simulink model "Suspension"  (R2019b)
settings: Solver=VariableStepAuto  StartTime=0.0  StopTime=10.0  RelTol=1e-3
values from neighbouring files (symbols this model uses):
  cfs = 1290    [Suspension_parameter.m]
  cft = 1000    [Suspension_parameter.m]
  crs = 1620    [Suspension_parameter.m]
  crt = 1000    [Suspension_parameter.m]
  iyy = 2460    [Suspension_parameter.m]
  kfs = 19960    [Suspension_parameter.m]
  kft = 175500    [Suspension_parameter.m]
  krs = 17500    [Suspension_parameter.m]
  krt = 175500    [Suspension_parameter.m]
  lf = 2.3    [Suspension_parameter.m]
  lr = 2.3    [Suspension_parameter.m]
  mc = 700    [Suspension_parameter.m]
  mf = 40    [Suspension_parameter.m]
  mr = 35.5    [Suspension_parameter.m]
libraries: simulink x4
(part 1 of 2)
settings Model: Creator=홍승표  LastModifiedBy=홍승표

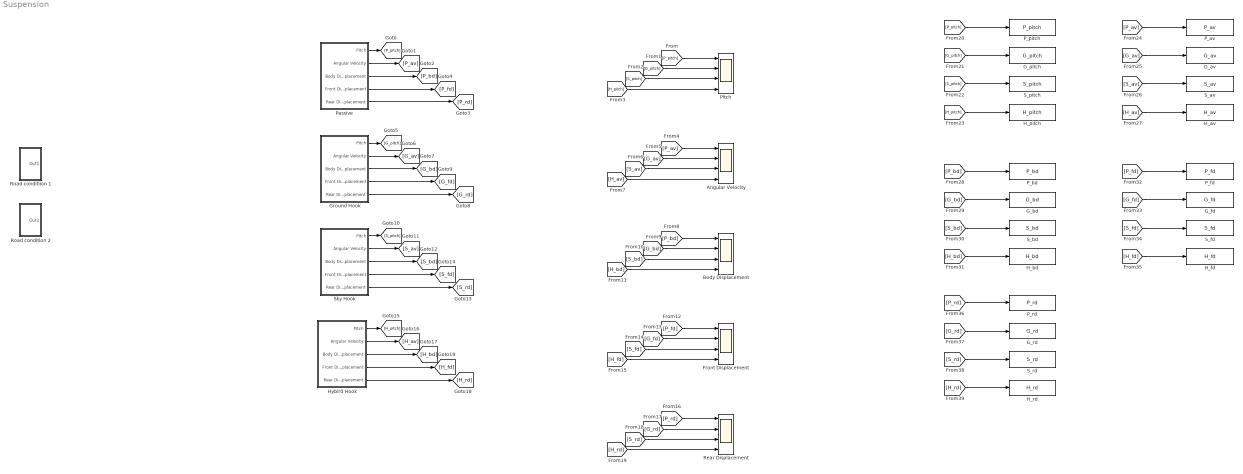
== system Suspension ==
  Angular Velocity : Scope  NumInputPorts=4
  Body Displacement : Scope  NumInputPorts=4
  Front Displacement : Scope  NumInputPorts=4
  G_av : ToWorkspace  VariableName=G_av  SampleTime=-1
  G_bd : ToWorkspace  VariableName=G_bd  SampleTime=-1
  G_fd : ToWorkspace  VariableName=G_fd  SampleTime=-1
  G_pitch : ToWorkspace  VariableName=G_pitch  SampleTime=-1
  G_rd : ToWorkspace  VariableName=G_rd  SampleTime=-1
  Ground Hook : Subsystem
  H_av : ToWorkspace  VariableName=H_av  SampleTime=-1
  H_bd : ToWorkspace  VariableName=H_bd  SampleTime=-1
  H_fd : ToWorkspace  VariableName=H_fd  SampleTime=-1
  H_pitch : ToWorkspace  VariableName=H_pitch  SampleTime=-1
  H_rd : ToWorkspace  VariableName=H_rd  SampleTime=-1
  Hybird Hook : Subsystem
  P_av : ToWorkspace  VariableName=P_av  SampleTime=-1
  P_bd : ToWorkspace  VariableName=P_bd  SampleTime=-1
  P_fd : ToWorkspace  VariableName=P_fd  SampleTime=-1
  P_pitch : ToWorkspace  VariableName=P_pitch  SampleTime=-1
  P_rd : ToWorkspace  VariableName=P_rd  SampleTime=-1
  Passive : Subsystem
  Pitch : Scope  NumInputPorts=4
  Rear Displacement : Scope  NumInputPorts=4
  Road conditiion 1 : Subsystem
  "Road condition 2 " : Subsystem
  S_av : ToWorkspace  VariableName=S_av  SampleTime=-1
  S_bd : ToWorkspace  VariableName=S_bd  SampleTime=-1
  S_fd : ToWorkspace  VariableName=S_fd  SampleTime=-1
  S_pitch : ToWorkspace  VariableName=S_pitch  SampleTime=-1
  S_rd : ToWorkspace  VariableName=S_rd  SampleTime=-1
  Sky Hook : Subsystem
  wires:
  Passive/1(Pitch) -> [P_pitch]
  Passive/2(Angular Velocity) -> [P_av]
  Passive/3(Body Displacement) -> [P_bd]
  Passive/4(Front Displacement) -> [P_fd]
  Passive/5(Rear Displacement) -> [P_rd]
  Ground Hook/2(Angular Velocity) -> [G_av]
  Ground Hook/5(Rear Displacement) -> [G_rd]
  Ground Hook/3(Body Displacement) -> [G_bd]
  Ground Hook/4(Front Displacement) -> [G_fd]
  Ground Hook/1(Pitch) -> [G_pitch]
  Sky Hook/4(Front Displacement) -> [S_fd]
  Sky Hook/1(Pitch) -> [S_pitch]
  Sky Hook/5(Rear Displacement) -> [S_rd]
  Sky Hook/2(Angular Velocity) -> [S_av]
  Sky Hook/3(Body Displacement) -> [S_bd]
  Hybird Hook/4(Front Displacement) -> [H_fd]
  Hybird Hook/1(Pitch) -> [H_pitch]
  Hybird Hook/5(Rear Displacement) -> [H_rd]
  Hybird Hook/2(Angular Velocity) -> [H_av]
  Hybird Hook/3(Body Displacement) -> [H_bd]
  [P_pitch] -> Pitch/1
  [G_pitch] -> Pitch/2
  [S_pitch] -> Pitch/3
  [H_pitch] -> Pitch/4
  [S_av] -> Angular Velocity/3
  [G_av] -> Angular Velocity/2
  [P_av] -> Angular Velocity/1
  [H_av] -> Angular Velocity/4
  [S_bd] -> Body Displacement/3
  [G_bd] -> Body Displacement/2
  [P_bd] -> Body Displacement/1
  [H_bd] -> Body Displacement/4
  [S_fd] -> Front Displacement/3
  [G_fd] -> Front Displacement/2
  [P_fd] -> Front Displacement/1
  [H_fd] -> Front Displacement/4
  [S_rd] -> Rear Displacement/3
  [G_rd] -> Rear Displacement/2
  [P_rd] -> Rear Displacement/1
  [H_rd] -> Rear Displacement/4
  [P_pitch] -> P_pitch/1
  [G_pitch] -> G_pitch/1
  [S_pitch] -> S_pitch/1
  [H_pitch] -> H_pitch/1
  [H_av] -> H_av/1
  [S_av] -> S_av/1
  [P_av] -> P_av/1
  [G_av] -> G_av/1
  [G_bd] -> G_bd/1
  [S_bd] -> S_bd/1
  [P_bd] -> P_bd/1
  [H_bd] -> H_bd/1
  [S_fd] -> S_fd/1
  [G_fd] -> G_fd/1
  [P_fd] -> P_fd/1
  [H_fd] -> H_fd/1
  [S_rd] -> S_rd/1
  [G_rd] -> G_rd/1
  [P_rd] -> P_rd/1
  [H_rd] -> H_rd/1

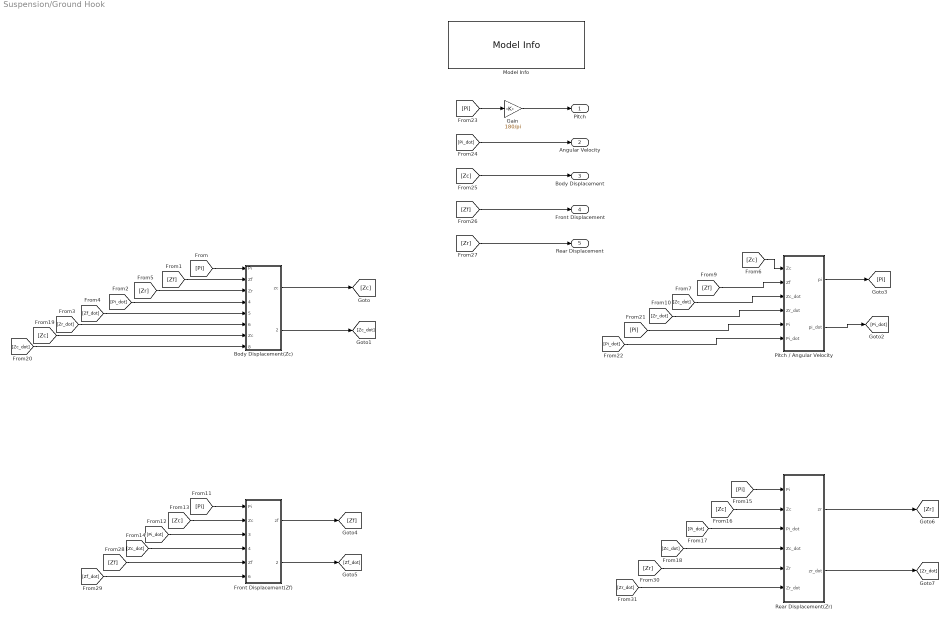
== system Suspension/Ground Hook ==
  Body Displacement(Zc) : Subsystem
  Front Displacement(Zf) : Subsystem
  Gain : Gain  Gain=180/pi
  Model Info : simulink/Model-Wide Utilities/Model Info  Frame=on  DisplayStringWithTags=Ground  HorizontalTextAlignment=Center  LeftAlignmentValue=0.5
  Pitch / Angular Velocity : Subsystem
  Rear Displacement(Zr) : Subsystem
  Pitch : Outport
  Angular Velocity : Outport  Port=2
  Body Displacement : Outport  Port=3
  Front Displacement : Outport  Port=4
  Rear Displacement : Outport  Port=5
  wires:
  [Pi_dot] -> Body Displacement(Zc)/4(Pi_dot)
  [Pi] -> Gain/1
  Front Displacement(Zf)/1(zf) -> [Zf]
  [Pi] -> Front Displacement(Zf)/1(Pi)
  Body Displacement(Zc)/1(zc) -> [Zc]
  [Pi_dot] -> Angular Velocity/1
  [Pi_dot] -> Rear Displacement(Zr)/3(Pi_dot)
  [Zr] -> Body Displacement(Zc)/3(Zr)
  [Zc_dot] -> Rear Displacement(Zr)/4(Zc_dot)
  [Zc] -> Body Displacement/1
  [Zr_dot] -> Body Displacement(Zc)/6(Zr_dot)
  Rear Displacement(Zr)/2(zr_dot) -> [Zr_dot]
  [Pi] -> Rear Displacement(Zr)/1(Pi)
  [Zf] -> Body Displacement(Zc)/2(Zf)
  [Zf_dot] -> Body Displacement(Zc)/5(Zf_dot)
  [Zc_dot] -> Front Displacement(Zf)/4(Zc_dot)
  Rear Displacement(Zr)/1(zr) -> [Zr]
  [Zc] -> Front Displacement(Zf)/2(Zc)
  [Zr] -> Rear Displacement/1
  Body Displacement(Zc)/2(zc_dot) -> [Zc_dot]
  Gain/1 -> Pitch/1
  [Zc] -> Rear Displacement(Zr)/2(Zc)
  [Zf] -> Front Displacement/1
  [Pi_dot] -> Front Displacement(Zf)/3(Pi_dot)
  Front Displacement(Zf)/2(zf_dot) -> [Zf_dot]
  [Pi] -> Body Displacement(Zc)/1(Pi)
  [Zc] -> Body Displacement(Zc)/7(Zc)
  [Zc_dot] -> Body Displacement(Zc)/8(Zc_dot)
  [Zf] -> Front Displacement(Zf)/5(Zf)
  [Zf_dot] -> Front Displacement(Zf)/6(Zf_dot)
  [Zr] -> Rear Displacement(Zr)/5(Zr)
  [Zr_dot] -> Rear Displacement(Zr)/6(Zr_dot)
  Pitch / Angular Velocity/1(pi) -> [Pi]
  [Pi] -> Pitch / Angular Velocity/5(Pi)
  [Zf] -> Pitch / Angular Velocity/2(Zf)
  [Zc_dot] -> Pitch / Angular Velocity/3(Zc_dot)
  [Zr_dot] -> Pitch / Angular Velocity/4(Zr_dot)
  Pitch / Angular Velocity/2(pi_dot) -> [Pi_dot]
  [Pi_dot] -> Pitch / Angular Velocity/6(Pi_dot)
  [Zc] -> Pitch / Angular Velocity/1(Zc)

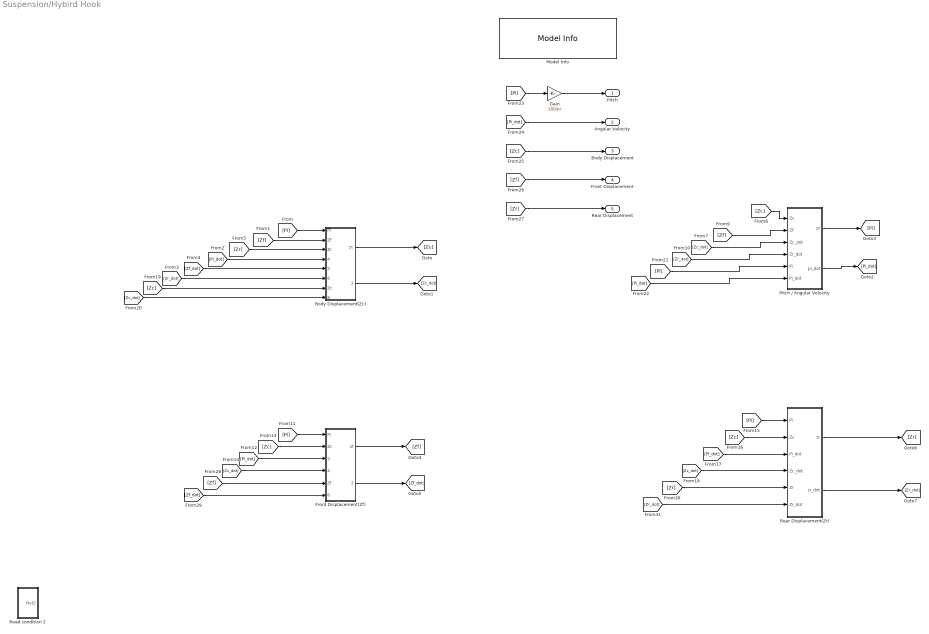
== system Suspension/Hybird Hook ==
  Body Displacement(Zc) : Subsystem
  Front Displacement(Zf) : Subsystem
  Gain : Gain  Gain=180/pi
  Model Info : simulink/Model-Wide Utilities/Model Info  Frame=on  DisplayStringWithTags=Hybrid  HorizontalTextAlignment=Center  LeftAlignmentValue=0.5
  Pitch / Angular Velocity : Subsystem
  Rear Displacement(Zr) : Subsystem
  "Road condition 2 " : Subsystem
  Pitch : Outport
  Angular Velocity : Outport  Port=2
  Body Displacement : Outport  Port=3
  Front Displacement : Outport  Port=4
  Rear Displacement : Outport  Port=5
  wires:
  [Pi_dot] -> Body Displacement(Zc)/4(Pi_dot)
  [Pi] -> Gain/1
  Front Displacement(Zf)/1(zf) -> [Zf]
  [Pi] -> Front Displacement(Zf)/1(Pi)
  Body Displacement(Zc)/1(zc) -> [Zc]
  [Pi_dot] -> Angular Velocity/1
  [Pi_dot] -> Rear Displacement(Zr)/3(Pi_dot)
  [Zr] -> Body Displacement(Zc)/3(Zr)
  [Zc_dot] -> Rear Displacement(Zr)/4(Zc_dot)
  [Zc] -> Body Displacement/1
  [Zr_dot] -> Body Displacement(Zc)/6(Zr_dot)
  Rear Displacement(Zr)/2(zr_dot) -> [Zr_dot]
  [Pi] -> Rear Displacement(Zr)/1(Pi)
  [Zf] -> Body Displacement(Zc)/2(Zf)
  [Zf_dot] -> Body Displacement(Zc)/5(Zf_dot)
  [Zc_dot] -> Front Displacement(Zf)/4(Zc_dot)
  Rear Displacement(Zr)/1(zr) -> [Zr]
  [Zc] -> Front Displacement(Zf)/2(Zc)
  [Zr] -> Rear Displacement/1
  Body Displacement(Zc)/2(zc_dot) -> [Zc_dot]
  Gain/1 -> Pitch/1
  [Zc] -> Rear Displacement(Zr)/2(Zc)
  [Zf] -> Front Displacement/1
  [Pi_dot] -> Front Displacement(Zf)/3(Pi_dot)
  Front Displacement(Zf)/2(zf_dot) -> [Zf_dot]
  [Pi] -> Body Displacement(Zc)/1(Pi)
  [Zc] -> Body Displacement(Zc)/7(Zc)
  [Zc_dot] -> Body Displacement(Zc)/8(Zc_dot)
  [Zf] -> Front Displacement(Zf)/5(Zf)
  [Zf_dot] -> Front Displacement(Zf)/6(Zf_dot)
  [Zr] -> Rear Displacement(Zr)/5(Zr)
  [Zr_dot] -> Rear Displacement(Zr)/6(Zr_dot)
  Pitch / Angular Velocity/1(pi) -> [Pi]
  [Pi] -> Pitch / Angular Velocity/5(Pi)
  [Zf] -> Pitch / Angular Velocity/2(Zf)
  [Zc_dot] -> Pitch / Angular Velocity/3(Zc_dot)
  [Zr_dot] -> Pitch / Angular Velocity/4(Zr_dot)
  Pitch / Angular Velocity/2(pi_dot) -> [Pi_dot]
  [Pi_dot] -> Pitch / Angular Velocity/6(Pi_dot)
  [Zc] -> Pitch / Angular Velocity/1(Zc)

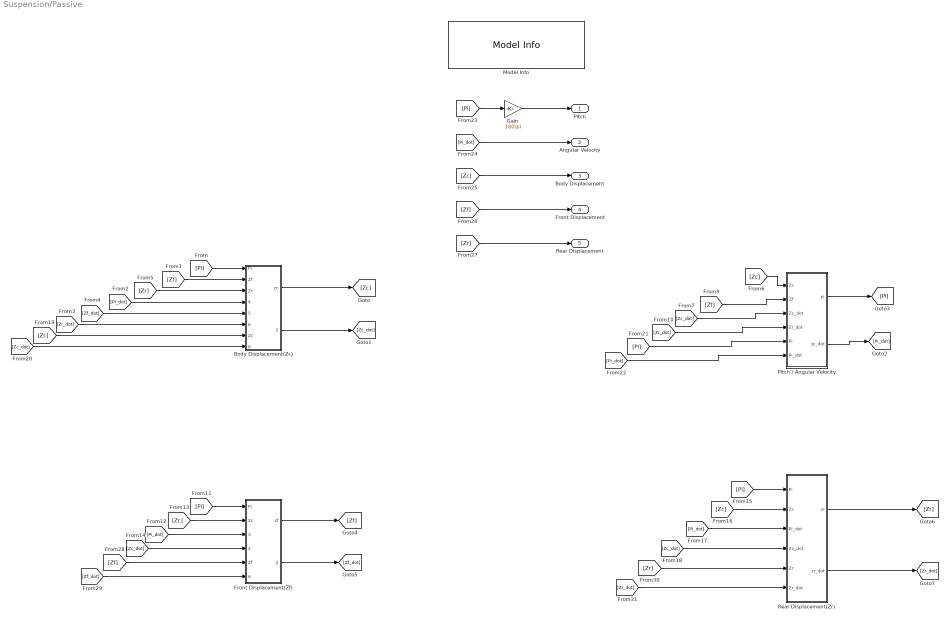
== system Suspension/Passive ==
  Body Displacement(Zc) : Subsystem
  Front Displacement(Zf) : Subsystem
  Gain : Gain  Gain=180/pi
  Model Info : simulink/Model-Wide Utilities/Model Info  Frame=on  DisplayStringWithTags=Passive  HorizontalTextAlignment=Center  LeftAlignmentValue=0.5
  Pitch / Angular Velocity : Subsystem
  Rear Displacement(Zr) : Subsystem
  Pitch : Outport
  Angular Velocity : Outport  Port=2
  Body Displacement : Outport  Port=3
  Front Displacement : Outport  Port=4
  Rear Displacement : Outport  Port=5
  wires:
  [Pi_dot] -> Body Displacement(Zc)/4(Pi_dot)
  [Pi] -> Gain/1
  Front Displacement(Zf)/1(zf) -> [Zf]
  [Pi] -> Front Displacement(Zf)/1(Pi)
  Body Displacement(Zc)/1(zc) -> [Zc]
  [Pi_dot] -> Angular Velocity/1
  [Pi_dot] -> Rear Displacement(Zr)/3(Pi_dot)
  [Zr] -> Body Displacement(Zc)/3(Zr)
  [Zc_dot] -> Rear Displacement(Zr)/4(Zc_dot)
  [Zc] -> Body Displacement/1
  [Zr_dot] -> Pitch / Angular Velocity/4(Zr_dot)
  [Zr_dot] -> Body Displacement(Zc)/6(Zr_dot)
  Rear Displacement(Zr)/2(zr_dot) -> [Zr_dot]
  [Pi] -> Rear Displacement(Zr)/1(Pi)
  [Zf] -> Body Displacement(Zc)/2(Zf)
  Pitch / Angular Velocity/1(pi) -> [Pi]
  [Zf_dot] -> Body Displacement(Zc)/5(Zf_dot)
  [Zc_dot] -> Front Displacement(Zf)/4(Zc_dot)
  Rear Displacement(Zr)/1(zr) -> [Zr]
  [Zc] -> Front Displacement(Zf)/2(Zc)
  [Zc] -> Pitch / Angular Velocity/1(Zc)
  [Zr] -> Rear Displacement/1
  Body Displacement(Zc)/2(zc_dot) -> [Zc_dot]
  Gain/1 -> Pitch/1
  [Zf] -> Pitch / Angular Velocity/2(Zf)
  [Zc_dot] -> Pitch / Angular Velocity/3(Zc_dot)
  [Zc] -> Rear Displacement(Zr)/2(Zc)
  [Zf] -> Front Displacement/1
  [Pi_dot] -> Front Displacement(Zf)/3(Pi_dot)
  Pitch / Angular Velocity/2(pi_dot) -> [Pi_dot]
  Front Displacement(Zf)/2(zf_dot) -> [Zf_dot]
  [Pi] -> Body Displacement(Zc)/1(Pi)
  [Zc] -> Body Displacement(Zc)/7(Zc)
  [Zc_dot] -> Body Displacement(Zc)/8(Zc_dot)
  [Pi] -> Pitch / Angular Velocity/5(Pi)
  [Pi_dot] -> Pitch / Angular Velocity/6(Pi_dot)
  [Zf] -> Front Displacement(Zf)/5(Zf)
  [Zf_dot] -> Front Displacement(Zf)/6(Zf_dot)
  [Zr] -> Rear Displacement(Zr)/5(Zr)
  [Zr_dot] -> Rear Displacement(Zr)/6(Zr_dot)

== system Suspension/Road conditiion 1 ==
  Gain : Gain
  Product : Product  Inputs=3
  Scope : Scope
  Signal Generator : SignalGenerator  Amplitude=0.15  Frequency=1.852  Units=rad/sec
  Step : Step  SampleTime=1.08
  Step1 : Step  Before=1  After=0  SampleTime=1.35
  Out1 : Outport
  wires:
  Gain/1 -> Out1/1
  Step1/1 -> Product/3
  Product/1 -> Gain/1, Scope/1
  Step/1 -> Product/2
  Signal Generator/1 -> Product/1

== system Suspension/Road condition 2  ==
  Product : Product  Inputs=3
  Saturation : Saturate  LowerLimit=0
  Scope : Scope
  Scope1 : Scope  NumInputPorts=3
  Signal Generator : SignalGenerator  Amplitude=0.15  Frequency=1.852
  Step : Step  SampleTime=1.08
  Step1 : Step  Before=1  After=0  SampleTime=4
  Out2 : Outport
  wires:
  Signal Generator/1 -> Scope1/1, Product/1
  Product/1 -> Out2/1, Saturation/1
  Step/1 -> Scope1/2, Product/2
  Step1/1 -> Scope1/3, Product/3
  Saturation/1 -> Scope/1

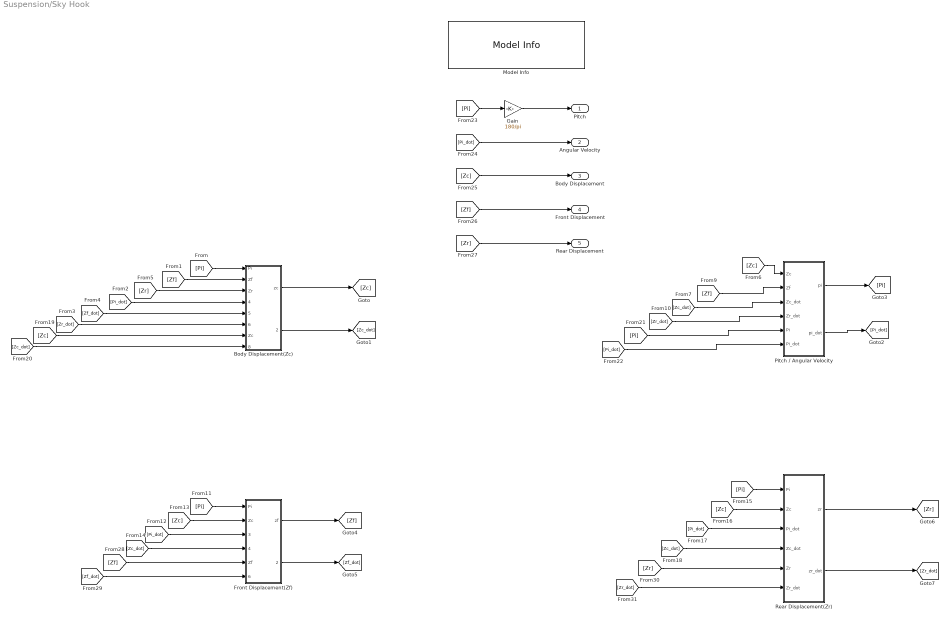
== system Suspension/Sky Hook ==
  Body Displacement(Zc) : Subsystem
  Front Displacement(Zf) : Subsystem
  Gain : Gain  Gain=180/pi
  Model Info : simulink/Model-Wide Utilities/Model Info  Frame=on  DisplayStringWithTags=Sky  HorizontalTextAlignment=Center  LeftAlignmentValue=0.5
  Pitch / Angular Velocity : Subsystem
  Rear Displacement(Zr) : Subsystem
  Pitch : Outport
  Angular Velocity : Outport  Port=2
  Body Displacement : Outport  Port=3
  Front Displacement : Outport  Port=4
  Rear Displacement : Outport  Port=5
  wires:
  [Pi_dot] -> Body Displacement(Zc)/4(Pi_dot)
  [Pi] -> Gain/1
  Front Displacement(Zf)/1(zf) -> [Zf]
  [Pi] -> Front Displacement(Zf)/1(Pi)
  Body Displacement(Zc)/1(zc) -> [Zc]
  [Pi_dot] -> Angular Velocity/1
  [Pi_dot] -> Rear Displacement(Zr)/3(Pi_dot)
  [Zr] -> Body Displacement(Zc)/3(Zr)
  [Zc_dot] -> Rear Displacement(Zr)/4(Zc_dot)
  [Zc] -> Body Displacement/1
  [Zr_dot] -> Body Displacement(Zc)/6(Zr_dot)
  Rear Displacement(Zr)/2(zr_dot) -> [Zr_dot]
  [Pi] -> Rear Displacement(Zr)/1(Pi)
  [Zf] -> Body Displacement(Zc)/2(Zf)
  [Zf_dot] -> Body Displacement(Zc)/5(Zf_dot)
  [Zc_dot] -> Front Displacement(Zf)/4(Zc_dot)
  Rear Displacement(Zr)/1(zr) -> [Zr]
  [Zc] -> Front Displacement(Zf)/2(Zc)
  [Zr] -> Rear Displacement/1
  Body Displacement(Zc)/2(zc_dot) -> [Zc_dot]
  Gain/1 -> Pitch/1
  [Zc] -> Rear Displacement(Zr)/2(Zc)
  [Zf] -> Front Displacement/1
  [Pi_dot] -> Front Displacement(Zf)/3(Pi_dot)
  Front Displacement(Zf)/2(zf_dot) -> [Zf_dot]
  [Pi] -> Body Displacement(Zc)/1(Pi)
  [Zc] -> Body Displacement(Zc)/7(Zc)
  [Zc_dot] -> Body Displacement(Zc)/8(Zc_dot)
  [Zf] -> Front Displacement(Zf)/5(Zf)
  [Zf_dot] -> Front Displacement(Zf)/6(Zf_dot)
  [Zr] -> Rear Displacement(Zr)/5(Zr)
  [Zr_dot] -> Rear Displacement(Zr)/6(Zr_dot)
  Pitch / Angular Velocity/1(pi) -> [Pi]
  [Pi] -> Pitch / Angular Velocity/5(Pi)
  [Zf] -> Pitch / Angular Velocity/2(Zf)
  [Zc_dot] -> Pitch / Angular Velocity/3(Zc_dot)
  [Zr_dot] -> Pitch / Angular Velocity/4(Zr_dot)
  Pitch / Angular Velocity/2(pi_dot) -> [Pi_dot]
  [Pi_dot] -> Pitch / Angular Velocity/6(Pi_dot)
  [Zc] -> Pitch / Angular Velocity/1(Zc)

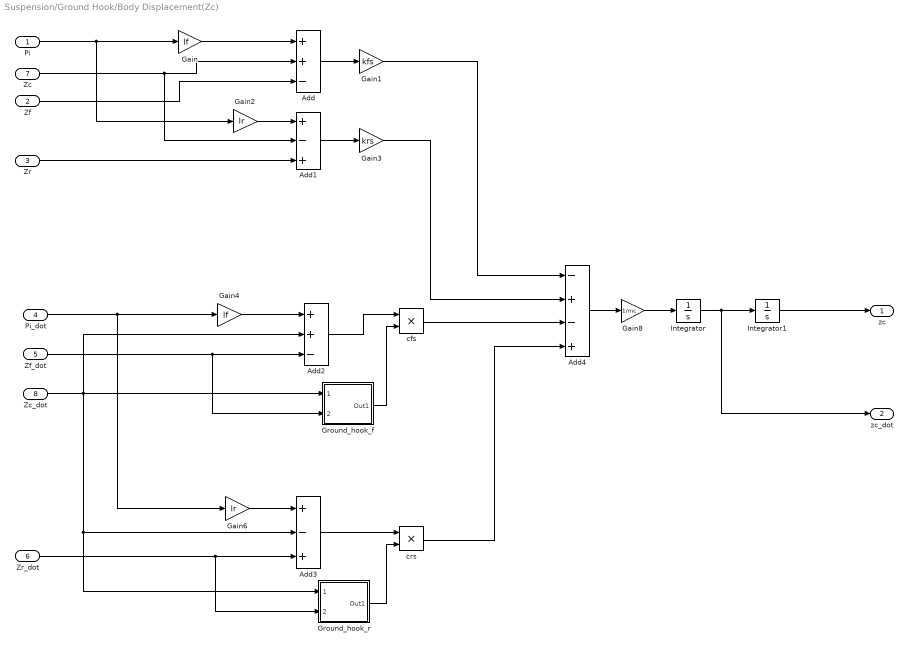
== system Suspension/Ground Hook/Body Displacement(Zc) ==
  Pi : Inport
  Zf : Inport  Port=2
  Zr : Inport  Port=3
  Pi_dot : Inport  Port=4
  Zf_dot : Inport  Port=5
  Zr_dot : Inport  Port=6
  Zc : Inport  Port=7
  Zc_dot : Inport  Port=8
  Add : Sum  Inputs=++-
  Add1 : Sum  Inputs=+-+
  Add2 : Sum  Inputs=++-
  Add3 : Sum  Inputs=+-+
  Add4 : Sum  Inputs=-+-+
  Gain : Gain  Gain=lf
  Gain1 : Gain  Gain=kfs
  Gain2 : Gain  Gain=lr
  Gain3 : Gain  Gain=krs
  Gain4 : Gain  Gain=lf
  Gain6 : Gain  Gain=lr
  Gain8 : Gain  Gain=1/mc
  Ground_hook_f : Subsystem
  Ground_hook_r : Subsystem
  Integrator : Integrator
  Integrator1 : Integrator
  cfs : Product
  crs : Product
  zc : Outport
  zc_dot : Outport  Port=2
  wires:
  Add/1 -> Gain1/1
  Add2/1 -> cfs/1
  Pi/1 -> Gain2/1, Gain/1
  Add4/1 -> Gain8/1
  Zr_dot/1 -> Ground_hook_r/2(Zr_dot), Add3/3
  Integrator/1 -> zc_dot/1, Integrator1/1
  Gain2/1 -> Add1/1
  Gain1/1 -> Add4/1
  Gain/1 -> Add/1
  Integrator1/1 -> zc/1
  crs/1 -> Add4/4
  Zr/1 -> Add1/3
  Add3/1 -> crs/1
  Zf_dot/1 -> Ground_hook_f/2(Zf_dot), Add2/3
  Gain6/1 -> Add3/1
  Gain3/1 -> Add4/2
  Pi_dot/1 -> Gain6/1, Gain4/1
  Gain4/1 -> Add2/1
  Add1/1 -> Gain3/1
  cfs/1 -> Add4/3
  Zf/1 -> Add/3
  Gain8/1 -> Integrator/1
  Ground_hook_f/1(Out1) -> cfs/2
  Ground_hook_r/1(Out1) -> crs/2
  Zc/1 -> Add1/2, Add/2
  Zc_dot/1 -> Add3/2, Ground_hook_r/1(Zc_dot), Ground_hook_f/1(Zc_dot), Add2/2

== system Suspension/Ground Hook/Front Displacement(Zf) ==
  Pi : Inport
  Zc : Inport  Port=2
  Pi_dot : Inport  Port=3
  Zc_dot : Inport  Port=4
  Zf : Inport  Port=5
  Zf_dot : Inport  Port=6
  Add10 : Sum  Inputs=++-
  Add11 : Sum  Inputs=++-
  Add12 : Sum  Inputs=+-
  Add13 : Sum  Inputs=+-
  Add14 : Sum  Inputs=++--
  Derivative : Derivative
  Gain22 : Gain  Gain=lf
  Gain23 : Gain  Gain=kfs
  Gain24 : Gain  Gain=lf
  Gain26 : Gain  Gain=kft
  Gain27 : Gain  Gain=cft
  Gain28 : Gain  Gain=1/mf
  Ground_hook_f : Subsystem
  Integrator4 : Integrator
  Integrator5 : Integrator
  Road conditiion 1 : Subsystem
  "Road condition 2 " : Subsystem
  cfs : Product
  zf : Outport
  zf_dot : Outport  Port=2
  wires:
  Gain28/1 -> Integrator4/1
  cfs/1 -> Add14/2
  Gain27/1 -> Add14/4
  Integrator4/1 -> zf_dot/1, Integrator5/1
  Add10/1 -> Gain23/1
  Integrator5/1 -> zf/1
  Gain24/1 -> Add11/1
  Gain23/1 -> Add14/1
  Add12/1 -> Gain27/1
  Gain26/1 -> Add14/3
  Gain22/1 -> Add10/1
  Add13/1 -> Gain26/1
  Add11/1 -> cfs/1
  Add14/1 -> Gain28/1
  Pi/1 -> Gain22/1
  Pi_dot/1 -> Gain24/1
  Zc/1 -> Add10/2
  Zc_dot/1 -> Ground_hook_f/1(Zc_dot), Add11/2
  Ground_hook_f/1(Out1) -> cfs/2
  Road conditiion 1/1(Out1) -> Add13/2, Derivative/1
  Derivative/1 -> Add12/2
  Zf/1 -> Add13/1, Add10/3
  Zf_dot/1 -> Add12/1, Add11/3, Ground_hook_f/2(Zf_dot)

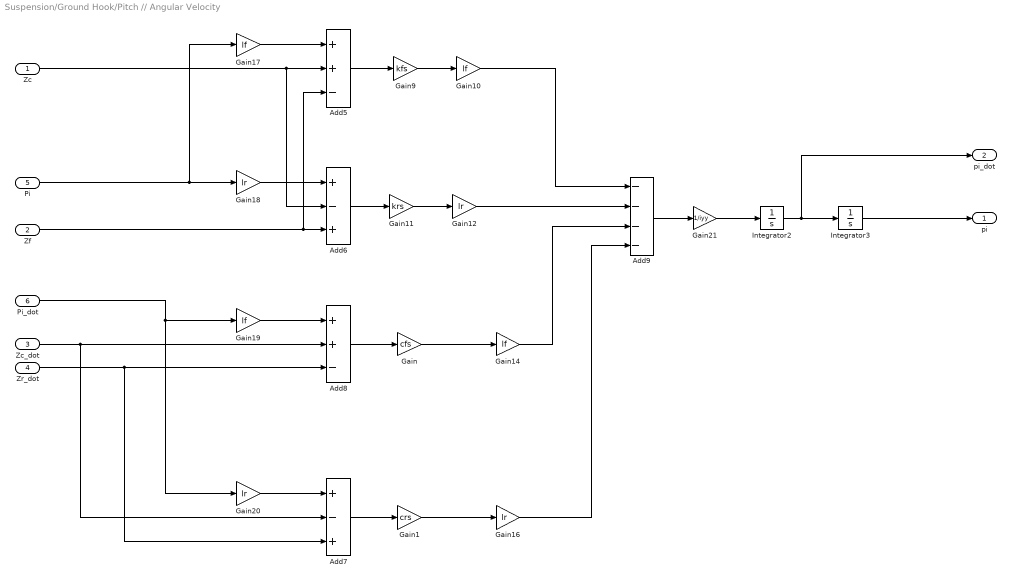
== system Suspension/Ground Hook/Pitch // Angular Velocity ==
  Zc : Inport
  Zf : Inport  Port=2
  Zc_dot : Inport  Port=3
  Zr_dot : Inport  Port=4
  Pi : Inport  Port=5
  Pi_dot : Inport  Port=6
  Add5 : Sum  Inputs=++-
  Add6 : Sum  Inputs=+-+
  Add7 : Sum  Inputs=+-+
  Add8 : Sum  Inputs=++-
  Add9 : Sum  Inputs=----
  Gain : Gain  Gain=cfs
  Gain1 : Gain  Gain=crs
  Gain{10,14,17,19} (4 alike) : Gain  Gain=lf
  Gain11 : Gain  Gain=krs
  Gain{12,16,18,20} (4 alike) : Gain  Gain=lr
  Gain21 : Gain  Gain=1/iyy
  Gain9 : Gain  Gain=kfs
  Integrator2 : Integrator
  Integrator3 : Integrator
  pi : Outport
  pi_dot : Outport  Port=2
  wires:
  Integrator3/1 -> pi/1
  Gain20/1 -> Add7/1
  Gain11/1 -> Gain12/1
  Gain9/1 -> Gain10/1
  Gain12/1 -> Add9/2
  Zc/1 -> Add6/2, Add5/2
  Add9/1 -> Gain21/1
  Gain17/1 -> Add5/1
  Zc_dot/1 -> Add7/2, Add8/2
  Gain16/1 -> Add9/4
  Zr_dot/1 -> Add7/3, Add8/3
  Integrator2/1 -> pi_dot/1, Integrator3/1
  Gain18/1 -> Add6/1
  Gain19/1 -> Add8/1
  Gain21/1 -> Integrator2/1
  Gain14/1 -> Add9/3
  Gain10/1 -> Add9/1
  Add5/1 -> Gain9/1
  Add6/1 -> Gain11/1
  Zf/1 -> Add5/3, Add6/3
  Pi_dot/1 -> Gain20/1, Gain19/1
  Pi/1 -> Gain17/1, Gain18/1
  Add8/1 -> Gain/1
  Gain/1 -> Gain14/1
  Add7/1 -> Gain1/1
  Gain1/1 -> Gain16/1

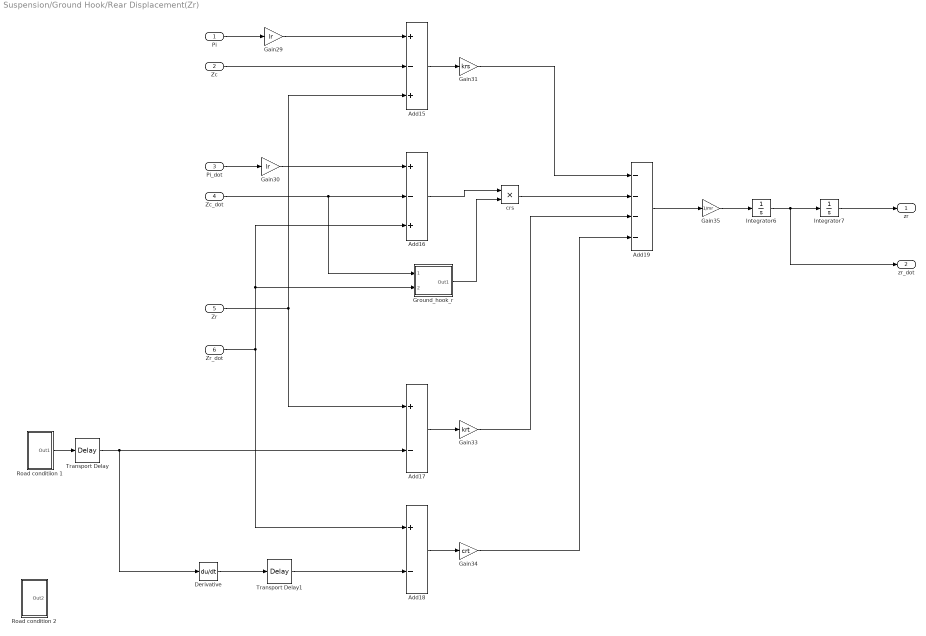
== system Suspension/Ground Hook/Rear Displacement(Zr) ==
  Pi : Inport
  Zc : Inport  Port=2
  Pi_dot : Inport  Port=3
  Zc_dot : Inport  Port=4
  Zr : Inport  Port=5
  Zr_dot : Inport  Port=6
  Add15 : Sum  Inputs=+-+
  Add16 : Sum  Inputs=+-+
  Add17 : Sum  Inputs=+-
  Add18 : Sum  Inputs=+-
  Add19 : Sum  Inputs=----
  Derivative : Derivative
  Gain29 : Gain  Gain=lr
  Gain30 : Gain  Gain=lr
  Gain31 : Gain  Gain=krs
  Gain33 : Gain  Gain=krt
  Gain34 : Gain  Gain=crt
  Gain35 : Gain  Gain=1/mr
  Ground_hook_r : Subsystem
  Integrator6 : Integrator
  Integrator7 : Integrator
  Road conditiion 1 : Subsystem
  "Road condition 2 " : Subsystem
  Transport Delay : TransportDelay  DelayTime=0.3
  Transport Delay1 : TransportDelay  DelayTime=0.3
  crs : Product
  zr : Outport
  zr_dot : Outport  Port=2
  wires:
  Gain35/1 -> Integrator6/1
  Zc_dot/1 -> Ground_hook_r/1(Zc_dot), Add16/2
  Integrator6/1 -> zr_dot/1, Integrator7/1
  Add17/1 -> Gain33/1
  Add15/1 -> Gain31/1
  Gain31/1 -> Add19/1
  Gain30/1 -> Add16/1
  Gain33/1 -> Add19/3
  Integrator7/1 -> zr/1
  Add16/1 -> crs/1
  Gain34/1 -> Add19/4
  Gain29/1 -> Add15/1
  Add18/1 -> Gain34/1
  Add19/1 -> Gain35/1
  crs/1 -> Add19/2
  Pi_dot/1 -> Gain30/1
  Pi/1 -> Gain29/1
  Zc/1 -> Add15/2
  Ground_hook_r/1(Out1) -> crs/2
  Transport Delay/1 -> Derivative/1, Add17/2
  Road conditiion 1/1(Out1) -> Transport Delay/1
  Zr/1 -> Add15/3, Add17/1
  Zr_dot/1 -> Add16/3, Ground_hook_r/2(Zr_dot), Add18/1
  Derivative/1 -> Transport Delay1/1
  Transport Delay1/1 -> Add18/2

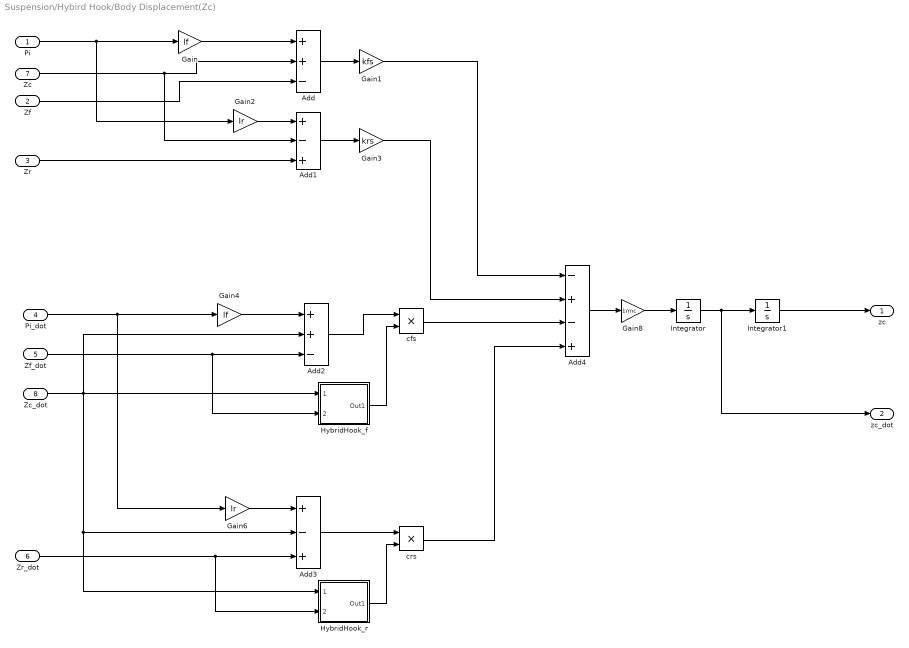
== system Suspension/Hybird Hook/Body Displacement(Zc) ==
  Pi : Inport
  Zf : Inport  Port=2
  Zr : Inport  Port=3
  Pi_dot : Inport  Port=4
  Zf_dot : Inport  Port=5
  Zr_dot : Inport  Port=6
  Zc : Inport  Port=7
  Zc_dot : Inport  Port=8
  Add : Sum  Inputs=++-
  Add1 : Sum  Inputs=+-+
  Add2 : Sum  Inputs=++-
  Add3 : Sum  Inputs=+-+
  Add4 : Sum  Inputs=-+-+
  Gain : Gain  Gain=lf
  Gain1 : Gain  Gain=kfs
  Gain2 : Gain  Gain=lr
  Gain3 : Gain  Gain=krs
  Gain4 : Gain  Gain=lf
  Gain6 : Gain  Gain=lr
  Gain8 : Gain  Gain=1/mc
  HybridHook_f : Subsystem
  HybridHook_r : Subsystem
  Integrator : Integrator
  Integrator1 : Integrator
  cfs : Product
  crs : Product
  zc : Outport
  zc_dot : Outport  Port=2
  wires:
  Add/1 -> Gain1/1
  Add2/1 -> cfs/1
  Pi/1 -> Gain2/1, Gain/1
  Add4/1 -> Gain8/1
  Zr_dot/1 -> HybridHook_r/2(Zr_dot), Add3/3
  Integrator/1 -> zc_dot/1, Integrator1/1
  Gain2/1 -> Add1/1
  Gain1/1 -> Add4/1
  Gain/1 -> Add/1
  Integrator1/1 -> zc/1
  crs/1 -> Add4/4
  Zr/1 -> Add1/3
  Add3/1 -> crs/1
  Zf_dot/1 -> HybridHook_f/2(Zf_dot), Add2/3
  Gain6/1 -> Add3/1
  Gain3/1 -> Add4/2
  Pi_dot/1 -> Gain6/1, Gain4/1
  Gain4/1 -> Add2/1
  Add1/1 -> Gain3/1
  cfs/1 -> Add4/3
  Zf/1 -> Add/3
  Gain8/1 -> Integrator/1
  HybridHook_f/1(Out1) -> cfs/2
  HybridHook_r/1(Out1) -> crs/2
  Zc/1 -> Add1/2, Add/2
  Zc_dot/1 -> HybridHook_f/1(Zc_dot), HybridHook_r/1(Zc_dot), Add3/2, Add2/2

== system Suspension/Hybird Hook/Front Displacement(Zf) ==
  Pi : Inport
  Zc : Inport  Port=2
  Pi_dot : Inport  Port=3
  Zc_dot : Inport  Port=4
  Zf : Inport  Port=5
  Zf_dot : Inport  Port=6
  Add10 : Sum  Inputs=++-
  Add11 : Sum  Inputs=++-
  Add12 : Sum  Inputs=+-
  Add13 : Sum  Inputs=+-
  Add14 : Sum  Inputs=++--
  Derivative : Derivative
  Gain22 : Gain  Gain=lf
  Gain23 : Gain  Gain=kfs
  Gain24 : Gain  Gain=lf
  Gain26 : Gain  Gain=kft
  Gain27 : Gain  Gain=cft
  Gain28 : Gain  Gain=1/mf
  HybridHook_f : Subsystem
  Integrator4 : Integrator
  Integrator5 : Integrator
  Road conditiion 1 : Subsystem
  "Road condition 2 " : Subsystem
  cfs : Product
  zf : Outport
  zf_dot : Outport  Port=2
  wires:
  Gain28/1 -> Integrator4/1
  cfs/1 -> Add14/2
  Gain27/1 -> Add14/4
  Integrator4/1 -> zf_dot/1, Integrator5/1
  Add10/1 -> Gain23/1
  Integrator5/1 -> zf/1
  Gain24/1 -> Add11/1
  Gain23/1 -> Add14/1
  Add12/1 -> Gain27/1
  Gain26/1 -> Add14/3
  Gain22/1 -> Add10/1
  Add13/1 -> Gain26/1
  Add11/1 -> cfs/1
  Add14/1 -> Gain28/1
  Pi/1 -> Gain22/1
  Pi_dot/1 -> Gain24/1
  Zc/1 -> Add10/2
  Zc_dot/1 -> HybridHook_f/1(Zc_dot), Add11/2
  HybridHook_f/1(Out1) -> cfs/2
  Road conditiion 1/1(Out1) -> Add13/2, Derivative/1
  Derivative/1 -> Add12/2
  Zf/1 -> Add13/1, Add10/3
  Zf_dot/1 -> Add12/1, HybridHook_f/2(Zf_dot), Add11/3

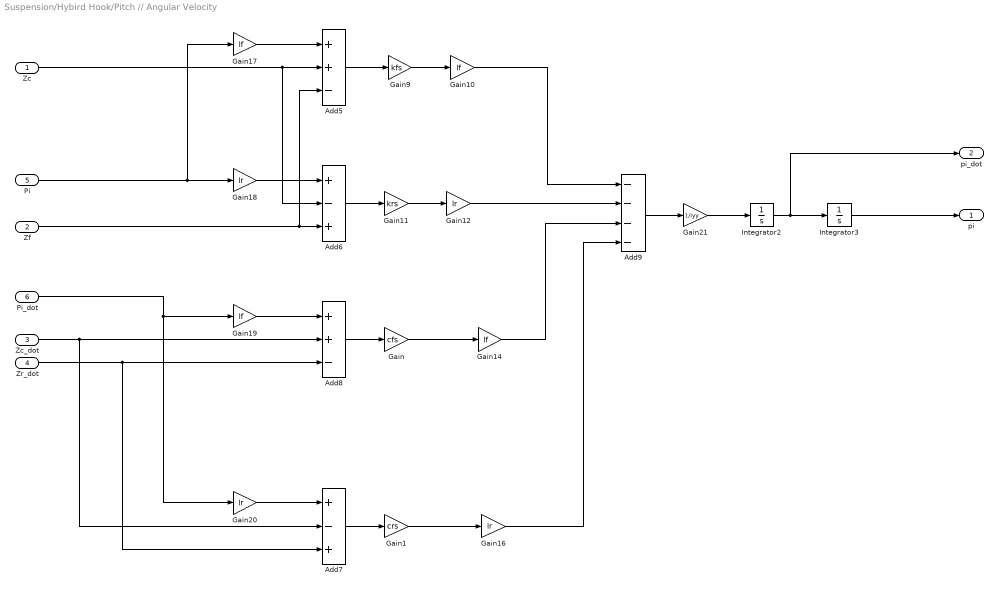
== system Suspension/Hybird Hook/Pitch // Angular Velocity ==
  Zc : Inport
  Zf : Inport  Port=2
  Zc_dot : Inport  Port=3
  Zr_dot : Inport  Port=4
  Pi : Inport  Port=5
  Pi_dot : Inport  Port=6
  Add5 : Sum  Inputs=++-
  Add6 : Sum  Inputs=+-+
  Add7 : Sum  Inputs=+-+
  Add8 : Sum  Inputs=++-
  Add9 : Sum  Inputs=----
  Gain : Gain  Gain=cfs
  Gain1 : Gain  Gain=crs
  Gain{10,14,17,19} (4 alike) : Gain  Gain=lf
  Gain11 : Gain  Gain=krs
  Gain{12,16,18,20} (4 alike) : Gain  Gain=lr
  Gain21 : Gain  Gain=1/iyy
  Gain9 : Gain  Gain=kfs
  Integrator2 : Integrator
  Integrator3 : Integrator
  pi : Outport
  pi_dot : Outport  Port=2
  wires:
  Integrator3/1 -> pi/1
  Gain20/1 -> Add7/1
  Gain11/1 -> Gain12/1
  Gain9/1 -> Gain10/1
  Gain12/1 -> Add9/2
  Zc/1 -> Add6/2, Add5/2
  Add9/1 -> Gain21/1
  Gain17/1 -> Add5/1
  Zc_dot/1 -> Add7/2, Add8/2
  Gain16/1 -> Add9/4
  Zr_dot/1 -> Add7/3, Add8/3
  Integrator2/1 -> pi_dot/1, Integrator3/1
  Gain18/1 -> Add6/1
  Gain19/1 -> Add8/1
  Gain21/1 -> Integrator2/1
  Gain14/1 -> Add9/3
  Gain10/1 -> Add9/1
  Add5/1 -> Gain9/1
  Add6/1 -> Gain11/1
  Zf/1 -> Add5/3, Add6/3
  Pi_dot/1 -> Gain20/1, Gain19/1
  Pi/1 -> Gain17/1, Gain18/1
  Add8/1 -> Gain/1
  Gain/1 -> Gain14/1
  Add7/1 -> Gain1/1
  Gain1/1 -> Gain16/1

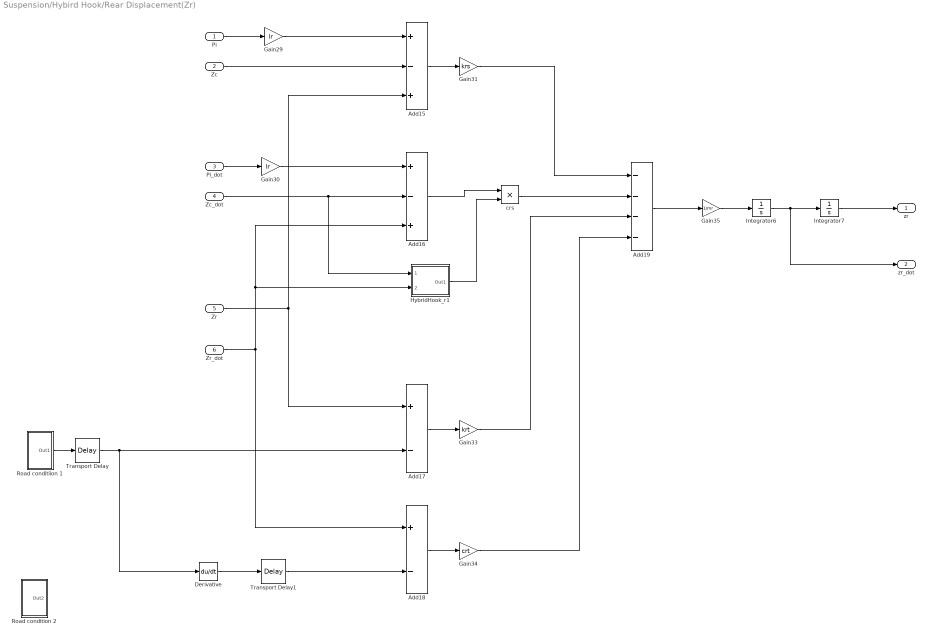
== system Suspension/Hybird Hook/Rear Displacement(Zr) ==
  Pi : Inport
  Zc : Inport  Port=2
  Pi_dot : Inport  Port=3
  Zc_dot : Inport  Port=4
  Zr : Inport  Port=5
  Zr_dot : Inport  Port=6
  Add15 : Sum  Inputs=+-+
  Add16 : Sum  Inputs=+-+
  Add17 : Sum  Inputs=+-
  Add18 : Sum  Inputs=+-
  Add19 : Sum  Inputs=----
  Derivative : Derivative
  Gain29 : Gain  Gain=lr
  Gain30 : Gain  Gain=lr
  Gain31 : Gain  Gain=krs
  Gain33 : Gain  Gain=krt
  Gain34 : Gain  Gain=crt
  Gain35 : Gain  Gain=1/mr
  HybridHook_r1 : Subsystem
  Integrator6 : Integrator
  Integrator7 : Integrator
  Road conditiion 1 : Subsystem
  "Road condition 2 " : Subsystem
  Transport Delay : TransportDelay  DelayTime=0.3
  Transport Delay1 : TransportDelay  DelayTime=0.3
  crs : Product
  zr : Outport
  zr_dot : Outport  Port=2
  wires:
  Gain35/1 -> Integrator6/1
  Zc_dot/1 -> HybridHook_r1/1(Zc_dot), Add16/2
  Integrator6/1 -> zr_dot/1, Integrator7/1
  Add17/1 -> Gain33/1
  Add15/1 -> Gain31/1
  Gain31/1 -> Add19/1
  Gain30/1 -> Add16/1
  Gain33/1 -> Add19/3
  Integrator7/1 -> zr/1
  Add16/1 -> crs/1
  Gain34/1 -> Add19/4
  Gain29/1 -> Add15/1
  Add18/1 -> Gain34/1
  Add19/1 -> Gain35/1
  crs/1 -> Add19/2
  Pi_dot/1 -> Gain30/1
  Pi/1 -> Gain29/1
  Zc/1 -> Add15/2
  HybridHook_r1/1(Out1) -> crs/2
  Transport Delay/1 -> Derivative/1, Add17/2
  Road conditiion 1/1(Out1) -> Transport Delay/1
  Zr/1 -> Add15/3, Add17/1
  Zr_dot/1 -> HybridHook_r1/2(Zr_dot), Add16/3, Add18/1
  Derivative/1 -> Transport Delay1/1
  Transport Delay1/1 -> Add18/2

== system Suspension/Hybird Hook/Road condition 2  ==
  Product : Product  Inputs=3
  Saturation : Saturate  LowerLimit=0
  Scope : Scope
  Signal Generator : SignalGenerator  Amplitude=0.07  Frequency=1.852
  Step : Step  SampleTime=1.08
  Step1 : Step  Before=1  After=0  SampleTime=4
  Out2 : Outport
  wires:
  Signal Generator/1 -> Product/1
  Product/1 -> Out2/1, Saturation/1
  Step/1 -> Product/2
  Step1/1 -> Product/3
  Saturation/1 -> Scope/1

== system Suspension/Passive/Body Displacement(Zc) ==
  Pi : Inport
  Zf : Inport  Port=2
  Zr : Inport  Port=3
  Pi_dot : Inport  Port=4
  Zf_dot : Inport  Port=5
  Zr_dot : Inport  Port=6
  Zc : Inport  Port=7
  Zc_dot : Inport  Port=8
  Add : Sum  Inputs=++-
  Add1 : Sum  Inputs=+-+
  Add2 : Sum  Inputs=++-
  Add3 : Sum  Inputs=+-+
  Add4 : Sum  Inputs=-+-+
  Gain : Gain  Gain=lf
  Gain1 : Gain  Gain=kfs
  Gain2 : Gain  Gain=lr
  Gain3 : Gain  Gain=krs
  Gain4 : Gain  Gain=lf
  Gain5 : Gain  Gain=cfs
  Gain6 : Gain  Gain=lr
  Gain7 : Gain  Gain=crs
  Gain8 : Gain  Gain=1/mc
  Integrator : Integrator
  Integrator1 : Integrator
  zc : Outport
  zc_dot : Outport  Port=2
  wires:
  Add/1 -> Gain1/1
  Pi/1 -> Gain2/1, Gain/1
  Add4/1 -> Gain8/1
  Zr_dot/1 -> Add3/3
  Integrator/1 -> zc_dot/1, Integrator1/1
  Gain2/1 -> Add1/1
  Gain1/1 -> Add4/1
  Gain/1 -> Add/1
  Integrator1/1 -> zc/1
  Zr/1 -> Add1/3
  Zf_dot/1 -> Add2/3
  Gain6/1 -> Add3/1
  Gain3/1 -> Add4/2
  Pi_dot/1 -> Gain6/1, Gain4/1
  Gain4/1 -> Add2/1
  Add1/1 -> Gain3/1
  Zf/1 -> Add/3
  Gain8/1 -> Integrator/1
  Zc/1 -> Add1/2, Add/2
  Zc_dot/1 -> Add3/2, Add2/2
  Add2/1 -> Gain5/1
  Gain5/1 -> Add4/3
  Add3/1 -> Gain7/1
  Gain7/1 -> Add4/4

== system Suspension/Passive/Front Displacement(Zf) ==
  Pi : Inport
  Zc : Inport  Port=2
  Pi_dot : Inport  Port=3
  Zc_dot : Inport  Port=4
  Zf : Inport  Port=5
  Zf_dot : Inport  Port=6
  Add10 : Sum  Inputs=++-
  Add11 : Sum  Inputs=++-
  Add12 : Sum  Inputs=+-
  Add13 : Sum  Inputs=+-
  Add14 : Sum  Inputs=++--
  Derivative : Derivative
  Gain : Gain  Gain=cfs
  Gain22 : Gain  Gain=lf
  Gain23 : Gain  Gain=kfs
  Gain24 : Gain  Gain=lf
  Gain26 : Gain  Gain=kft
  Gain27 : Gain  Gain=cft
  Gain28 : Gain  Gain=1/mf
  Integrator4 : Integrator
  Integrator5 : Integrator
  Road conditiion 1 : Subsystem
  "Road condition 2 " : Subsystem
  zf : Outport
  zf_dot : Outport  Port=2
  wires:
  Gain28/1 -> Integrator4/1
  Gain27/1 -> Add14/4
  Integrator4/1 -> zf_dot/1, Integrator5/1
  Add10/1 -> Gain23/1
  Integrator5/1 -> zf/1
  Gain24/1 -> Add11/1
  Gain23/1 -> Add14/1
  Add12/1 -> Gain27/1
  Gain26/1 -> Add14/3
  Gain22/1 -> Add10/1
  Add13/1 -> Gain26/1
  Add14/1 -> Gain28/1
  Pi/1 -> Gain22/1
  Pi_dot/1 -> Gain24/1
  Zc/1 -> Add10/2
  Zc_dot/1 -> Add11/2
  Road conditiion 1/1(Out1) -> Add13/2, Derivative/1
  Derivative/1 -> Add12/2
  Zf/1 -> Add13/1, Add10/3
  Zf_dot/1 -> Add12/1, Add11/3
  Add11/1 -> Gain/1
  Gain/1 -> Add14/2

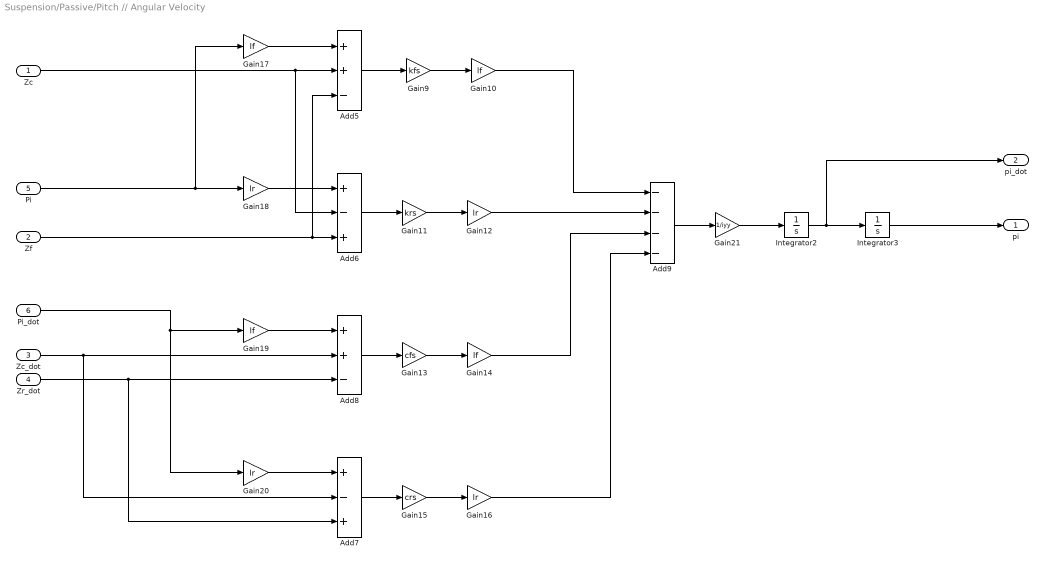
== system Suspension/Passive/Pitch // Angular Velocity ==
  Zc : Inport
  Zf : Inport  Port=2
  Zc_dot : Inport  Port=3
  Zr_dot : Inport  Port=4
  Pi : Inport  Port=5
  Pi_dot : Inport  Port=6
  Add5 : Sum  Inputs=++-
  Add6 : Sum  Inputs=+-+
  Add7 : Sum  Inputs=+-+
  Add8 : Sum  Inputs=++-
  Add9 : Sum  Inputs=----
  Gain{10,14,17,19} (4 alike) : Gain  Gain=lf
  Gain11 : Gain  Gain=krs
  Gain{12,16,18,20} (4 alike) : Gain  Gain=lr
  Gain13 : Gain  Gain=cfs
  Gain15 : Gain  Gain=crs
  Gain21 : Gain  Gain=1/iyy
  Gain9 : Gain  Gain=kfs
  Integrator2 : Integrator
  Integrator3 : Integrator
  pi : Outport
  pi_dot : Outport  Port=2
  wires:
  Integrator3/1 -> pi/1
  Gain20/1 -> Add7/1
  Gain11/1 -> Gain12/1
  Gain9/1 -> Gain10/1
  Gain12/1 -> Add9/2
  Zc/1 -> Add6/2, Add5/2
  Add9/1 -> Gain21/1
  Gain15/1 -> Gain16/1
  Gain17/1 -> Add5/1
  Zc_dot/1 -> Add7/2, Add8/2
  Gain13/1 -> Gain14/1
  Gain16/1 -> Add9/4
  Zr_dot/1 -> Add7/3, Add8/3
  Integrator2/1 -> pi_dot/1, Integrator3/1
  Gain18/1 -> Add6/1
  Gain19/1 -> Add8/1
  Gain21/1 -> Integrator2/1
  Gain14/1 -> Add9/3
  Gain10/1 -> Add9/1
  Add5/1 -> Gain9/1
  Add8/1 -> Gain13/1
  Add7/1 -> Gain15/1
  Add6/1 -> Gain11/1
  Zf/1 -> Add5/3, Add6/3
  Pi_dot/1 -> Gain20/1, Gain19/1
  Pi/1 -> Gain17/1, Gain18/1

== system Suspension/Passive/Rear Displacement(Zr) ==
  Pi : Inport
  Zc : Inport  Port=2
  Pi_dot : Inport  Port=3
  Zc_dot : Inport  Port=4
  Zr : Inport  Port=5
  Zr_dot : Inport  Port=6
  Add15 : Sum  Inputs=+-+
  Add16 : Sum  Inputs=+-+
  Add17 : Sum  Inputs=+-
  Add18 : Sum  Inputs=+-
  Add19 : Sum  Inputs=----
  Derivative : Derivative
  Gain : Gain  Gain=crs
  Gain29 : Gain  Gain=lr
  Gain30 : Gain  Gain=lr
  Gain31 : Gain  Gain=krs
  Gain33 : Gain  Gain=krt
  Gain34 : Gain  Gain=crt
  Gain35 : Gain  Gain=1/mr
  Integrator6 : Integrator
  Integrator7 : Integrator
  Road conditiion 1 : Subsystem
  "Road condition 2 " : Subsystem
  Transport Delay : TransportDelay
  Transport Delay1 : TransportDelay  DelayTime=0.3
  zr : Outport
  zr_dot : Outport  Port=2
  wires:
  Gain35/1 -> Integrator6/1
  Zc_dot/1 -> Add16/2
  Integrator6/1 -> zr_dot/1, Integrator7/1
  Add17/1 -> Gain33/1
  Add15/1 -> Gain31/1
  Gain31/1 -> Add19/1
  Gain30/1 -> Add16/1
  Gain33/1 -> Add19/3
  Integrator7/1 -> zr/1
  Gain34/1 -> Add19/4
  Gain29/1 -> Add15/1
  Add18/1 -> Gain34/1
  Add19/1 -> Gain35/1
  Pi_dot/1 -> Gain30/1
  Pi/1 -> Gain29/1
  Zc/1 -> Add15/2
  Road conditiion 1/1(Out1) -> Transport Delay/1
  Derivative/1 -> Transport Delay1/1
  Zr/1 -> Add15/3, Add17/1
  Zr_dot/1 -> Add16/3, Add18/1
  Add16/1 -> Gain/1
  Gain/1 -> Add19/2
  Transport Delay/1 -> Derivative/1, Add17/2
  Transport Delay1/1 -> Add18/2

== system Suspension/Sky Hook/Body Displacement(Zc) ==
  Pi : Inport
  Zf : Inport  Port=2
  Zr : Inport  Port=3
  Pi_dot : Inport  Port=4
  Zf_dot : Inport  Port=5
  Zr_dot : Inport  Port=6
  Zc : Inport  Port=7
  Zc_dot : Inport  Port=8
  Add : Sum  Inputs=++-
  Add1 : Sum  Inputs=+-+
  Add2 : Sum  Inputs=++-
  Add3 : Sum  Inputs=+-+
  Add4 : Sum  Inputs=-+-+
  Gain : Gain  Gain=lf
  Gain1 : Gain  Gain=kfs
  Gain2 : Gain  Gain=lr
  Gain3 : Gain  Gain=krs
  Gain4 : Gain  Gain=lf
  Gain6 : Gain  Gain=lr
  Gain8 : Gain  Gain=1/mc
  Integrator : Integrator
  Integrator1 : Integrator
  Sky Hook_f : Subsystem
  Sky Hook_r : Subsystem
  cfs : Product
  crs : Product
  zc : Outport
  zc_dot : Outport  Port=2
  wires:
  Add/1 -> Gain1/1
  Add2/1 -> cfs/1
  Pi/1 -> Gain2/1, Gain/1
  Add4/1 -> Gain8/1
  Zr_dot/1 -> Sky Hook_r/2(Zr_dot), Add3/3
  Integrator/1 -> zc_dot/1, Integrator1/1
  Gain2/1 -> Add1/1
  Gain1/1 -> Add4/1
  Gain/1 -> Add/1
  Integrator1/1 -> zc/1
  crs/1 -> Add4/4
  Zr/1 -> Add1/3
  Add3/1 -> crs/1
  Zf_dot/1 -> Sky Hook_f/2(Zf_dot), Add2/3
  Gain6/1 -> Add3/1
  Gain3/1 -> Add4/2
  Pi_dot/1 -> Gain6/1, Gain4/1
  Gain4/1 -> Add2/1
  Add1/1 -> Gain3/1
  cfs/1 -> Add4/3
  Zf/1 -> Add/3
  Gain8/1 -> Integrator/1
  Sky Hook_f/1(Out1) -> cfs/2
  Sky Hook_r/1(Out1) -> crs/2
  Zc/1 -> Add1/2, Add/2
  Zc_dot/1 -> Sky Hook_f/1(Zc_dot), Sky Hook_r/1(Zc_dot), Add3/2, Add2/2

== system Suspension/Sky Hook/Front Displacement(Zf) ==
  Pi : Inport
  Zc : Inport  Port=2
  Pi_dot : Inport  Port=3
  Zc_dot : Inport  Port=4
  Zf : Inport  Port=5
  Zf_dot : Inport  Port=6
  Add10 : Sum  Inputs=++-
  Add11 : Sum  Inputs=++-
  Add12 : Sum  Inputs=+-
  Add13 : Sum  Inputs=+-
  Add14 : Sum  Inputs=++--
  Derivative : Derivative
  Gain22 : Gain  Gain=lf
  Gain23 : Gain  Gain=kfs
  Gain24 : Gain  Gain=lf
  Gain26 : Gain  Gain=kft
  Gain27 : Gain  Gain=cft
  Gain28 : Gain  Gain=1/mf
  Integrator4 : Integrator
  Integrator5 : Integrator
  Road conditiion 1 : Subsystem
  "Road condition 2 " : Subsystem
  Sky Hook_f : Subsystem
  cfs : Product
  zf : Outport
  zf_dot : Outport  Port=2
  wires:
  Gain28/1 -> Integrator4/1
  cfs/1 -> Add14/2
  Gain27/1 -> Add14/4
  Integrator4/1 -> zf_dot/1, Integrator5/1
  Add10/1 -> Gain23/1
  Integrator5/1 -> zf/1
  Gain24/1 -> Add11/1
  Gain23/1 -> Add14/1
  Add12/1 -> Gain27/1
  Gain26/1 -> Add14/3
  Gain22/1 -> Add10/1
  Add13/1 -> Gain26/1
  Add11/1 -> cfs/1
  Add14/1 -> Gain28/1
  Pi/1 -> Gain22/1
  Pi_dot/1 -> Gain24/1
  Zc/1 -> Add10/2
  Zc_dot/1 -> Sky Hook_f/1(Zc_dot), Add11/2
  Sky Hook_f/1(Out1) -> cfs/2
  Road conditiion 1/1(Out1) -> Add13/2, Derivative/1
  Derivative/1 -> Add12/2
  Zf/1 -> Add13/1, Add10/3
  Zf_dot/1 -> Add12/1, Sky Hook_f/2(Zf_dot), Add11/3

== system Suspension/Sky Hook/Pitch // Angular Velocity ==
  Zc : Inport
  Zf : Inport  Port=2
  Zc_dot : Inport  Port=3
  Zr_dot : Inport  Port=4
  Pi : Inport  Port=5
  Pi_dot : Inport  Port=6
  Add5 : Sum  Inputs=++-
  Add6 : Sum  Inputs=+-+
  Add7 : Sum  Inputs=+-+
  Add8 : Sum  Inputs=++-
  Add9 : Sum  Inputs=----
  Gain : Gain  Gain=cfs
  Gain1 : Gain  Gain=crs
  Gain{10,14,17,19} (4 alike) : Gain  Gain=lf
  Gain11 : Gain  Gain=krs
  Gain{12,16,18,20} (4 alike) : Gain  Gain=lr
  Gain21 : Gain  Gain=1/iyy
  Gain9 : Gain  Gain=kfs
  Integrator2 : Integrator
  Integrator3 : Integrator
  pi : Outport
  pi_dot : Outport  Port=2
  wires:
  Integrator3/1 -> pi/1
  Gain20/1 -> Add7/1
  Gain11/1 -> Gain12/1
  Gain9/1 -> Gain10/1
  Gain12/1 -> Add9/2
  Zc/1 -> Add6/2, Add5/2
  Add9/1 -> Gain21/1
  Gain17/1 -> Add5/1
  Zc_dot/1 -> Add7/2, Add8/2
  Gain16/1 -> Add9/4
  Zr_dot/1 -> Add7/3, Add8/3
  Integrator2/1 -> pi_dot/1, Integrator3/1
  Gain18/1 -> Add6/1
  Gain19/1 -> Add8/1
  Gain21/1 -> Integrator2/1
  Gain14/1 -> Add9/3
  Gain10/1 -> Add9/1
  Add5/1 -> Gain9/1
  Add6/1 -> Gain11/1
  Zf/1 -> Add5/3, Add6/3
  Pi_dot/1 -> Gain20/1, Gain19/1
  Pi/1 -> Gain17/1, Gain18/1
  Add8/1 -> Gain/1
  Add7/1 -> Gain1/1
  Gain/1 -> Gain14/1
  Gain1/1 -> Gain16/1

== system Suspension/Sky Hook/Rear Displacement(Zr) ==
  Pi : Inport
  Zc : Inport  Port=2
  Pi_dot : Inport  Port=3
  Zc_dot : Inport  Port=4
  Zr : Inport  Port=5
  Zr_dot : Inport  Port=6
  Add15 : Sum  Inputs=+-+
  Add16 : Sum  Inputs=+-+
  Add17 : Sum  Inputs=+-
  Add18 : Sum  Inputs=+-
  Add19 : Sum  Inputs=----
  Derivative : Derivative
  Gain29 : Gain  Gain=lr
  Gain30 : Gain  Gain=lr
  Gain31 : Gain  Gain=krs
  Gain33 : Gain  Gain=krt
  Gain34 : Gain  Gain=crt
  Gain35 : Gain  Gain=1/mr
  Integrator6 : Integrator
  Integrator7 : Integrator
  Road conditiion 1 : Subsystem
  "Road condition 2 " : Subsystem
  Sky Hook_r1 : Subsystem
  Transport Delay : TransportDelay  DelayTime=0.3
  Transport Delay1 : TransportDelay  DelayTime=0.3
  crs : Product
  zr : Outport
  zr_dot : Outport  Port=2
  wires:
  Gain35/1 -> Integrator6/1
  Zc_dot/1 -> Sky Hook_r1/1(Zc_dot), Add16/2
  Integrator6/1 -> zr_dot/1, Integrator7/1
  Add17/1 -> Gain33/1
  Add15/1 -> Gain31/1
  Gain31/1 -> Add19/1
  Gain30/1 -> Add16/1
  Gain33/1 -> Add19/3
  Integrator7/1 -> zr/1
  Add16/1 -> crs/1
  Gain34/1 -> Add19/4
  Gain29/1 -> Add15/1
  Add18/1 -> Gain34/1
  Add19/1 -> Gain35/1
  crs/1 -> Add19/2
  Pi_dot/1 -> Gain30/1
  Pi/1 -> Gain29/1
  Zc/1 -> Add15/2
  Sky Hook_r1/1(Out1) -> crs/2
  Transport Delay/1 -> Derivative/1, Add17/2
  Road conditiion 1/1(Out1) -> Transport Delay/1
  Derivative/1 -> Transport Delay1/1
  Zr/1 -> Add15/3, Add17/1
  Zr_dot/1 -> Sky Hook_r1/2(Zr_dot), Add16/3, Add18/1
  Transport Delay1/1 -> Add18/2

== system Suspension/Ground Hook/Body Displacement(Zc)/Ground_hook_f ==
  Zc_dot : Inport
  Zf_dot : Inport  Port=2
  Add5 : Sum  Inputs=+-
  Constant : Constant  Value=2838
  Constant1 : Constant  Value=258
  Gain9 : Gain  Gain=-1
  If : If  IfExpression=u1 >= 0  ZeroCross=off
  Merge : Merge
  Product : Product
  Switch Case Action Subsystem : Subsystem  TreatAsAtomicUnit=on
  Switch Case Action Subsystem2 : Subsystem  TreatAsAtomicUnit=on
  Out1 : Outport
  wires:
  Zf_dot/1 -> Gain9/1, Add5/2
  If/1 -> Switch Case Action Subsystem/Action
  Constant1/1 -> Switch Case Action Subsystem2/1(In1)
  Product/1 -> If/1
  Add5/1 -> Product/1
  Switch Case Action Subsystem2/1(Out1) -> Merge/2
  Gain9/1 -> Product/2
  If/2 -> Switch Case Action Subsystem2/Action
  Constant/1 -> Switch Case Action Subsystem/1(1)
  Switch Case Action Subsystem/1(Csa) -> Merge/1
  Merge/1 -> Out1/1
  Zc_dot/1 -> Add5/1

== system Suspension/Ground Hook/Body Displacement(Zc)/Ground_hook_r ==
  Zc_dot : Inport
  Zr_dot : Inport  Port=2
  Add5 : Sum  Inputs=+-
  Constant : Constant  Value=2838
  Constant1 : Constant  Value=258
  Gain9 : Gain  Gain=-1
  If : If  IfExpression=u1 >= 0  ZeroCross=off
  Merge : Merge
  Product : Product
  Switch Case Action Subsystem : Subsystem  TreatAsAtomicUnit=on
  Switch Case Action Subsystem2 : Subsystem  TreatAsAtomicUnit=on
  Out1 : Outport
  wires:
  Zr_dot/1 -> Gain9/1, Add5/2
  If/1 -> Switch Case Action Subsystem/Action
  Constant1/1 -> Switch Case Action Subsystem2/1(In1)
  Product/1 -> If/1
  Add5/1 -> Product/1
  Switch Case Action Subsystem2/1(Out1) -> Merge/2
  Gain9/1 -> Product/2
  If/2 -> Switch Case Action Subsystem2/Action
  Constant/1 -> Switch Case Action Subsystem/1(1)
  Switch Case Action Subsystem/1(Csa) -> Merge/1
  Merge/1 -> Out1/1
  Zc_dot/1 -> Add5/1

== system Suspension/Ground Hook/Front Displacement(Zf)/Ground_hook_f ==
  Zc_dot : Inport
  Zf_dot : Inport  Port=2
  Add5 : Sum  Inputs=+-
  Constant : Constant  Value=2838
  Constant1 : Constant  Value=258
  Gain9 : Gain  Gain=-1
  If : If  IfExpression=u1 >= 0  ZeroCross=off
  Merge : Merge
  Product : Product
  Switch Case Action Subsystem : Subsystem  TreatAsAtomicUnit=on
  Switch Case Action Subsystem2 : Subsystem  TreatAsAtomicUnit=on
  Out1 : Outport
  wires:
  Zf_dot/1 -> Gain9/1, Add5/2
  If/1 -> Switch Case Action Subsystem/Action
  Constant1/1 -> Switch Case Action Subsystem2/1(In1)
  Product/1 -> If/1
  Add5/1 -> Product/1
  Switch Case Action Subsystem2/1(Out1) -> Merge/2
  Gain9/1 -> Product/2
  If/2 -> Switch Case Action Subsystem2/Action
  Constant/1 -> Switch Case Action Subsystem/1(1)
  Switch Case Action Subsystem/1(Csa) -> Merge/1
  Merge/1 -> Out1/1
  Zc_dot/1 -> Add5/1

== system Suspension/Ground Hook/Front Displacement(Zf)/Road conditiion 1 ==
  Gain : Gain
  Product : Product  Inputs=3
  Scope : Scope
  Signal Generator : SignalGenerator  Amplitude=0.15  Frequency=1.852  Units=rad/sec
  Step : Step  SampleTime=1.08
  Step1 : Step  Before=1  After=0  SampleTime=1.35
  Out1 : Outport
  wires:
  Gain/1 -> Out1/1
  Step1/1 -> Product/3
  Product/1 -> Gain/1, Scope/1
  Step/1 -> Product/2
  Signal Generator/1 -> Product/1

== system Suspension/Ground Hook/Front Displacement(Zf)/Road condition 2  ==
  Product : Product  Inputs=3
  Saturation : Saturate  LowerLimit=0
  Scope : Scope
  Signal Generator : SignalGenerator  Amplitude=0.15  Frequency=1.852
  Step : Step  SampleTime=1.08
  Step1 : Step  Before=1  After=0  SampleTime=4
  Out2 : Outport
  wires:
  Signal Generator/1 -> Product/1
  Product/1 -> Out2/1, Saturation/1
  Step/1 -> Product/2
  Step1/1 -> Product/3
  Saturation/1 -> Scope/1

== system Suspension/Ground Hook/Rear Displacement(Zr)/Ground_hook_r ==
  Zc_dot : Inport
  Zr_dot : Inport  Port=2
  Add5 : Sum  Inputs=+-
  Constant : Constant  Value=2838
  Constant1 : Constant  Value=258
  Gain9 : Gain  Gain=-1
  If : If  IfExpression=u1 >= 0  ZeroCross=off
  Merge : Merge
  Product : Product
  Switch Case Action Subsystem : Subsystem  TreatAsAtomicUnit=on
  Switch Case Action Subsystem2 : Subsystem  TreatAsAtomicUnit=on
  Out1 : Outport
  wires:
  Zr_dot/1 -> Gain9/1, Add5/2
  If/1 -> Switch Case Action Subsystem/Action
  Constant1/1 -> Switch Case Action Subsystem2/1(In1)
  Product/1 -> If/1
  Add5/1 -> Product/1
  Switch Case Action Subsystem2/1(Out1) -> Merge/2
  Gain9/1 -> Product/2
  If/2 -> Switch Case Action Subsystem2/Action
  Constant/1 -> Switch Case Action Subsystem/1(1)
  Switch Case Action Subsystem/1(Csa) -> Merge/1
  Merge/1 -> Out1/1
  Zc_dot/1 -> Add5/1

== system Suspension/Ground Hook/Rear Displacement(Zr)/Road conditiion 1 ==
  Gain : Gain
  Product : Product  Inputs=3
  Scope : Scope
  Scope1 : Scope  NumInputPorts=3
  Signal Generator : SignalGenerator  Amplitude=0.15  Frequency=1.852  Units=rad/sec
  Step : Step  SampleTime=1.08
  Step1 : Step  Before=1  After=0  SampleTime=1.35
  Out1 : Outport
  wires:
  Gain/1 -> Out1/1
  Step1/1 -> Scope1/3, Product/3
  Product/1 -> Gain/1, Scope/1
  Step/1 -> Scope1/2, Product/2
  Signal Generator/1 -> Scope1/1, Product/1

== system Suspension/Ground Hook/Rear Displacement(Zr)/Road condition 2  ==
  Product : Product  Inputs=3
  Saturation : Saturate  LowerLimit=0
  Scope : Scope
  Signal Generator : SignalGenerator  Amplitude=0.15  Frequency=1.852
  Step : Step  SampleTime=1.08
  Step1 : Step  Before=1  After=0  SampleTime=4
  Out2 : Outport
  wires:
  Signal Generator/1 -> Product/1
  Product/1 -> Out2/1, Saturation/1
  Step/1 -> Product/2
  Step1/1 -> Product/3
  Saturation/1 -> Scope/1

== system Suspension/Hybird Hook/Body Displacement(Zc)/HybridHook_f ==
  Zc_dot : Inport
  Zf_dot : Inport  Port=2
  Add1 : Sum
  GroundHook : Subsystem
  SkyHook : Subsystem
  Out1 : Outport
  wires:
  GroundHook/1(Out1) -> Add1/1
  Add1/1 -> Out1/1
  SkyHook/1(Out1) -> Add1/2
  Zf_dot/1 -> GroundHook/2(In2), SkyHook/2(In2)
  Zc_dot/1 -> GroundHook/1(In1), SkyHook/1(In1)

== system Suspension/Hybird Hook/Body Displacement(Zc)/HybridHook_r ==
  Zc_dot : Inport
  Zr_dot : Inport  Port=2
  Add1 : Sum
  GroundHook : Subsystem
  SkyHook : Subsystem
  Out1 : Outport
  wires:
  GroundHook/1(Out1) -> Add1/1
  Add1/1 -> Out1/1
  SkyHook/1(Out1) -> Add1/2
  Zr_dot/1 -> GroundHook/2(In2), SkyHook/2(In2)
  Zc_dot/1 -> GroundHook/1(In1), SkyHook/1(In1)

== system Suspension/Hybird Hook/Front Displacement(Zf)/HybridHook_f ==
  Zc_dot : Inport
  Zf_dot : Inport  Port=2
  Add1 : Sum
  GroundHook : Subsystem
  SkyHook : Subsystem
  Out1 : Outport
  wires:
  GroundHook/1(Out1) -> Add1/1
  Add1/1 -> Out1/1
  SkyHook/1(Out1) -> Add1/2
  Zf_dot/1 -> GroundHook/2(In2), SkyHook/2(In2)
  Zc_dot/1 -> GroundHook/1(In1), SkyHook/1(In1)

== system Suspension/Hybird Hook/Front Displacement(Zf)/Road conditiion 1 ==
  Gain : Gain
  Product : Product  Inputs=3
  Scope : Scope
  Signal Generator : SignalGenerator  Amplitude=0.15  Frequency=1.852  Units=rad/sec
  Step : Step  SampleTime=1.08
  Step1 : Step  Before=1  After=0  SampleTime=1.35
  Out1 : Outport
  wires:
  Gain/1 -> Out1/1
  Step1/1 -> Product/3
  Product/1 -> Gain/1, Scope/1
  Step/1 -> Product/2
  Signal Generator/1 -> Product/1

== system Suspension/Hybird Hook/Front Displacement(Zf)/Road condition 2  ==
  Product : Product  Inputs=3
  Saturation : Saturate  LowerLimit=0
  Scope : Scope
  Signal Generator : SignalGenerator  Amplitude=0.15  Frequency=1.852  Units=rad/sec
  Step : Step  SampleTime=1.08
  Step1 : Step  Before=1  After=0  SampleTime=4
  Out2 : Outport
  wires:
  Signal Generator/1 -> Product/1
  Product/1 -> Out2/1, Saturation/1
  Step/1 -> Product/2
  Step1/1 -> Product/3
  Saturation/1 -> Scope/1

== system Suspension/Hybird Hook/Rear Displacement(Zr)/HybridHook_r1 ==
  Zc_dot : Inport
  Zr_dot : Inport  Port=2
  Add1 : Sum
  GroundHook : Subsystem
  SkyHook : Subsystem
  Out1 : Outport
  wires:
  GroundHook/1(Out1) -> Add1/1
  Add1/1 -> Out1/1
  SkyHook/1(Out1) -> Add1/2
  Zr_dot/1 -> GroundHook/2(In2), SkyHook/2(In2)
  Zc_dot/1 -> GroundHook/1(In1), SkyHook/1(In1)

== system Suspension/Hybird Hook/Rear Displacement(Zr)/Road conditiion 1 ==
  Gain : Gain
  Product : Product  Inputs=3
  Scope : Scope
  Signal Generator : SignalGenerator  Amplitude=0.15  Frequency=1.852  Units=rad/sec
  Step : Step  SampleTime=1.08
  Step1 : Step  Before=1  After=0  SampleTime=1.35
  Out1 : Outport
  wires:
  Gain/1 -> Out1/1
  Step1/1 -> Product/3
  Product/1 -> Gain/1, Scope/1
  Step/1 -> Product/2
  Signal Generator/1 -> Product/1

== system Suspension/Hybird Hook/Rear Displacement(Zr)/Road condition 2  ==
  Product : Product  Inputs=3
  Saturation : Saturate  LowerLimit=0
  Scope : Scope
  Signal Generator : SignalGenerator  Amplitude=0.15  Frequency=1.852  Units=rad/sec
  Step : Step  SampleTime=1.08
  Step1 : Step  Before=1  After=0  SampleTime=4
  Out2 : Outport
  wires:
  Signal Generator/1 -> Product/1
  Product/1 -> Out2/1, Saturation/1
  Step/1 -> Product/2
  Step1/1 -> Product/3
  Saturation/1 -> Scope/1

== system Suspension/Passive/Front Displacement(Zf)/Road conditiion 1 ==
  Gain : Gain
  Product : Product  Inputs=3
  Scope : Scope
  Signal Generator : SignalGenerator  Amplitude=0.15  Frequency=1.852  Units=rad/sec
  Step : Step  SampleTime=1.08
  Step1 : Step  Before=1  After=0  SampleTime=1.35
  Out1 : Outport
  wires:
  Gain/1 -> Out1/1
  Step1/1 -> Product/3
  Product/1 -> Gain/1, Scope/1
  Step/1 -> Product/2
  Signal Generator/1 -> Product/1

== system Suspension/Passive/Front Displacement(Zf)/Road condition 2  ==
  Product : Product  Inputs=3
  Saturation : Saturate  LowerLimit=0
  Scope : Scope
  Signal Generator : SignalGenerator  Amplitude=0.15  Frequency=1.852
  Step : Step  SampleTime=1.08
  Step1 : Step  Before=1  After=0  SampleTime=4
  Out2 : Outport
  wires:
  Signal Generator/1 -> Product/1
  Product/1 -> Out2/1, Saturation/1
  Step/1 -> Product/2
  Step1/1 -> Product/3
  Saturation/1 -> Scope/1

== system Suspension/Passive/Rear Displacement(Zr)/Road conditiion 1 ==
  Gain : Gain
  Product : Product  Inputs=3
  Scope : Scope
  Signal Generator : SignalGenerator  Amplitude=0.15  Frequency=1.852  Units=rad/sec
  Step : Step  SampleTime=1.08
  Step1 : Step  Before=1  After=0  SampleTime=1.35
  Out1 : Outport
  wires:
  Gain/1 -> Out1/1
  Step1/1 -> Product/3
  Product/1 -> Gain/1, Scope/1
  Step/1 -> Product/2
  Signal Generator/1 -> Product/1

== system Suspension/Passive/Rear Displacement(Zr)/Road condition 2  ==
  Product : Product  Inputs=3
  Saturation : Saturate  LowerLimit=0
  Scope : Scope
  Signal Generator : SignalGenerator  Amplitude=0.15  Frequency=1.852  Units=rad/sec
  Step : Step  SampleTime=1.08
  Step1 : Step  Before=1  After=0  SampleTime=4
  Out2 : Outport
  wires:
  Signal Generator/1 -> Product/1
  Product/1 -> Out2/1, Saturation/1
  Step/1 -> Product/2
  Step1/1 -> Product/3
  Saturation/1 -> Scope/1

== system Suspension/Sky Hook/Body Displacement(Zc)/Sky Hook_f ==
  Zc_dot : Inport
  Zf_dot : Inport  Port=2
  Add : Sum  Inputs=+-
  Constant : Constant  Value=2838
  Constant1 : Constant  Value=258
  If : If  IfExpression=u1 >= 0  ZeroCross=off
  Merge : Merge
  Product : Product
  Switch Case Action Subsystem : Subsystem  TreatAsAtomicUnit=on
  Switch Case Action Subsystem1 : Subsystem  TreatAsAtomicUnit=on
  Out1 : Outport
  wires:
  Constant1/1 -> Switch Case Action Subsystem1/1(In1)
  Zc_dot/1 -> Product/1, Add/1
  Switch Case Action Subsystem/1(Out1) -> Merge/1
  Switch Case Action Subsystem1/1(Out1) -> Merge/2
  Add/1 -> Product/2
  Product/1 -> If/1
  If/2 -> Switch Case Action Subsystem1/Action
  If/1 -> Switch Case Action Subsystem/Action
  Constant/1 -> Switch Case Action Subsystem/1(In1)
  Zf_dot/1 -> Add/2
  Merge/1 -> Out1/1

== system Suspension/Sky Hook/Body Displacement(Zc)/Sky Hook_r ==
  Zc_dot : Inport
  Zr_dot : Inport  Port=2
  Add : Sum  Inputs=+-
  Constant : Constant  Value=2838
  Constant1 : Constant  Value=258
  If : If  IfExpression=u1 >= 0  ZeroCross=off
  Merge : Merge
  Product : Product
  Switch Case Action Subsystem : Subsystem  TreatAsAtomicUnit=on
  Switch Case Action Subsystem1 : Subsystem  TreatAsAtomicUnit=on
  Out1 : Outport
  wires:
  Constant1/1 -> Switch Case Action Subsystem1/1(In1)
  Zc_dot/1 -> Product/1, Add/1
  Switch Case Action Subsystem/1(Out1) -> Merge/1
  Switch Case Action Subsystem1/1(Out1) -> Merge/2
  Add/1 -> Product/2
  Product/1 -> If/1
  If/2 -> Switch Case Action Subsystem1/Action
  If/1 -> Switch Case Action Subsystem/Action
  Constant/1 -> Switch Case Action Subsystem/1(In1)
  Zr_dot/1 -> Add/2
  Merge/1 -> Out1/1

== system Suspension/Sky Hook/Front Displacement(Zf)/Road conditiion 1 ==
  Gain : Gain
  Product : Product  Inputs=3
  Scope : Scope
  Signal Generator : SignalGenerator  Amplitude=0.15  Frequency=1.852  Units=rad/sec
  Step : Step  SampleTime=1.08
  Step1 : Step  Before=1  After=0  SampleTime=1.35
  Out1 : Outport
  wires:
  Gain/1 -> Out1/1
  Step1/1 -> Product/3
  Product/1 -> Gain/1, Scope/1
  Step/1 -> Product/2
  Signal Generator/1 -> Product/1
